simulink model "VCU_CS75_12_27_test_log"  (R2014a)
settings: Solver=FixedStepDiscrete  StartTime=0.0  StopTime=25  FixedStep=0.0005  RelTol=1e-3
undefined symbols (not defined in the file or in its folder): ecucoder_acal, ErrorSumMax1, ErrorSumMax2, ErrorSumMax3, I1, I2, I3, I_SW01_L, LaterlAngleCommand, LDW, Log_ErrorSumMax1, Log_ErrorSumMax2, Log_I1, Log_I2, Log_P1, Log_P2, Log_Takeover, P1, P2, P3, RemoteAcc, RemoteAcclPosition
libraries: simulink x927, ec5744lib x40
(part 24 of 31)

== system VCU_CS75_12_27_test_log/长安CS75底盘程序，20ms一次/Input/CAN0_Rx/a1_211/ReceiveMessages/Subsystem/a1 ==
  input : Inport
  Demux : Demux  Outputs=8
  SCS_Ad : Sum
  SCS_Convert : DataTypeConversion  OutDataTypeStr=uint32
  SCS_F : Gain
  SCS_L : simulink/Logic and Bit Operations/Bitwise Operator  logicop=AND  UseBitMask=on  BitMask=8  BitMaskRealWorld=Stored Integer
  SCS_O : Constant  Value=0  OutDataTypeStr=single
  SCS_S : ArithShift  BitShiftNumber=3
  SCS_Sub : Subsystem
  SCS_sat : Saturate  UpperLimit=1  LowerLimit=0
  SCScv : DataTypeConversion
  Vx_Ad : Sum
  Vx_Convert : DataTypeConversion  OutDataTypeStr=uint32
  Vx_F : Gain  Gain=0.00610360875867857
  Vx_L : simulink/Logic and Bit Operations/Bitwise Operator  logicop=AND  UseBitMask=on  BitMask=65535  BitMaskRealWorld=Stored Integer
  Vx_O : Constant  Value=-200  OutDataTypeStr=single
  Vx_S : ArithShift
  Vx_Sub : Subsystem
  Vx_sat : Saturate  UpperLimit=200  LowerLimit=-200
  Vxcv : DataTypeConversion
  Vxinput8_Ad : Sum
  Vxinput8_C : Constant  Value=256
  Vxinput8_P : Product
  cones_count_actual_Ad : Sum
  cones_count_actual_Convert : DataTypeConversion  OutDataTypeStr=uint32
  cones_count_actual_F : Gain
  cones_count_actual_L : simulink/Logic and Bit Operations/Bitwise Operator  logicop=AND  UseBitMask=on  BitMask=255  BitMaskRealWorld=Stored Integer
  cones_count_actual_O : Constant  Value=0  OutDataTypeStr=single
  cones_count_actual_S : ArithShift
  cones_count_actual_Sub : Subsystem
  cones_count_actual_sat : Saturate  UpperLimit=255  LowerLimit=0
  cones_count_actualcv : DataTypeConversion
  cones_count_all_Ad : Sum
  cones_count_all_Convert : DataTypeConversion  OutDataTypeStr=uint32
  cones_count_all_F : Gain
  cones_count_all_L : simulink/Logic and Bit Operations/Bitwise Operator  logicop=AND  UseBitMask=on  BitMask=255  BitMaskRealWorld=Stored Integer
  cones_count_all_O : Constant  Value=0  OutDataTypeStr=single
  cones_count_all_S : ArithShift
  cones_count_all_Sub : Subsystem
  cones_count_all_sat : Saturate  UpperLimit=255  LowerLimit=0
  cones_count_allcv : DataTypeConversion
  finish_Ad : Sum
  finish_Convert : DataTypeConversion  OutDataTypeStr=uint32
  finish_F : Gain
  finish_L : simulink/Logic and Bit Operations/Bitwise Operator  logicop=AND  UseBitMask=on  BitMask=4  BitMaskRealWorld=Stored Integer
  finish_O : Constant  Value=0  OutDataTypeStr=single
  finish_S : ArithShift  BitShiftNumber=2
  finish_Sub : Subsystem
  finish_sat : Saturate  UpperLimit=1  LowerLimit=0
  finishcv : DataTypeConversion
  mission_Ad : Sum
  mission_Convert : DataTypeConversion  OutDataTypeStr=uint32
  mission_F : Gain
  mission_L : simulink/Logic and Bit Operations/Bitwise Operator  logicop=AND  UseBitMask=on  BitMask=240  BitMaskRealWorld=Stored Integer
  mission_O : Constant  Value=0  OutDataTypeStr=single
  mission_S : ArithShift  BitShiftNumber=4
  mission_Sub : Subsystem
  mission_sat : Saturate  UpperLimit=7  LowerLimit=0
  missioncv : DataTypeConversion
  tap_Ad : Sum
  tap_Convert : DataTypeConversion  OutDataTypeStr=uint32
  tap_F : Gain
  tap_L : simulink/Logic and Bit Operations/Bitwise Operator  logicop=AND  UseBitMask=on  BitMask=3  BitMaskRealWorld=Stored Integer
  tap_O : Constant  Value=0  OutDataTypeStr=single
  tap_S : ArithShift
  tap_Sub : Subsystem
  tap_sat : Saturate  UpperLimit=3  LowerLimit=0
  tapcv : DataTypeConversion
  target_steering_Ad : Sum
  target_steering_Convert : DataTypeConversion  OutDataTypeStr=uint32
  target_steering_F : Gain  Gain=0.0488400488400488
  target_steering_L : simulink/Logic and Bit Operations/Bitwise Operator  logicop=AND  UseBitMask=on  BitMask=4095  BitMaskRealWorld=Stored Integer
  target_steering_O : Constant  Value=-100  OutDataTypeStr=single
  target_steering_S : ArithShift
  target_steering_Sub : Subsystem
  target_steering_sat : Saturate  UpperLimit=99.9999999999998  LowerLimit=-100
  target_steeringcv : DataTypeConversion
  target_steeringinput2_Ad : Sum
  target_steeringinput2_C : Constant  Value=256
  target_steeringinput2_P : Product
  throttlevbrake_position_Ad : Sum
  throttlevbrake_position_Convert : DataTypeConversion  OutDataTypeStr=uint32
  throttlevbrake_position_F : Gain  Gain=0.0488400488400488
  throttlevbrake_position_L : simulink/Logic and Bit Operations/Bitwise Operator  logicop=AND  UseBitMask=on  BitMask=65520  BitMaskRealWorld=Stored Integer
  throttlevbrake_position_O : Constant  Value=-100  OutDataTypeStr=single
  throttlevbrake_position_S : ArithShift  BitShiftNumber=4
  throttlevbrake_position_Sub : Subsystem
  throttlevbrake_position_sat : Saturate  UpperLimit=100  LowerLimit=-100
  throttlevbrake_positioncv : DataTypeConversion
  throttlevbrake_positioninput3_Ad : Sum
  throttlevbrake_positioninput3_C : Constant  Value=256
  throttlevbrake_positioninput3_P : Product
  Vx_Out : Outport
  mission_Out : Outport  Port=2
  SCS_Out : Outport  Port=3
  finish_Out : Outport  Port=4
  tap_Out : Outport  Port=5
  cones_count_all_Out : Outport  Port=6
  cones_count_actual_Out : Outport  Port=7
  throttlevbrake_position_Out : Outport  Port=8
  target_steering_Out : Outport  Port=9
  wires:
  Vx_F/1 -> Vx_Ad/1
  Vx_O/1 -> Vx_Ad/2
  Vx_Ad/1 -> Vx_sat/1
  Vx_sat/1 -> Vx_Out/1
  Demux/8 -> Vxinput8_P/1
  Vxinput8_C/1 -> Vxinput8_P/2
  Vxinput8_P/1 -> Vxinput8_Ad/1
  Demux/7 -> Vxinput8_Ad/2
  Vxinput8_Ad/1 -> Vx_Sub/1(In1)
  Vx_Sub/1(Out1) -> Vx_Convert/1
  Vx_Convert/1 -> Vx_L/1
  Vx_L/1 -> Vx_S/1
  Vx_S/1 -> Vxcv/1
  Vxcv/1 -> Vx_F/1
  mission_F/1 -> mission_Ad/1
  mission_O/1 -> mission_Ad/2
  mission_Ad/1 -> mission_sat/1
  mission_sat/1 -> mission_Out/1
  Demux/6 -> mission_Sub/1(In1), SCS_Sub/1(In1), finish_Sub/1(In1), tap_Sub/1(In1)
  mission_Sub/1(Out1) -> mission_Convert/1
  mission_Convert/1 -> mission_L/1
  mission_L/1 -> mission_S/1
  mission_S/1 -> missioncv/1
  missioncv/1 -> mission_F/1
  SCS_F/1 -> SCS_Ad/1
  SCS_O/1 -> SCS_Ad/2
  SCS_Ad/1 -> SCS_sat/1
  SCS_sat/1 -> SCS_Out/1
  SCS_Sub/1(Out1) -> SCS_Convert/1
  SCS_Convert/1 -> SCS_L/1
  SCS_L/1 -> SCS_S/1
  SCS_S/1 -> SCScv/1
  SCScv/1 -> SCS_F/1
  finish_F/1 -> finish_Ad/1
  finish_O/1 -> finish_Ad/2
  finish_Ad/1 -> finish_sat/1
  finish_sat/1 -> finish_Out/1
  finish_Sub/1(Out1) -> finish_Convert/1
  finish_Convert/1 -> finish_L/1
  finish_L/1 -> finish_S/1
  finish_S/1 -> finishcv/1
  finishcv/1 -> finish_F/1
  tap_F/1 -> tap_Ad/1
  tap_O/1 -> tap_Ad/2
  tap_Ad/1 -> tap_sat/1
  tap_sat/1 -> tap_Out/1
  tap_Sub/1(Out1) -> tap_Convert/1
  tap_Convert/1 -> tap_L/1
  tap_L/1 -> tap_S/1
  tap_S/1 -> tapcv/1
  tapcv/1 -> tap_F/1
  cones_count_all_F/1 -> cones_count_all_Ad/1
  cones_count_all_O/1 -> cones_count_all_Ad/2
  cones_count_all_Ad/1 -> cones_count_all_sat/1
  cones_count_all_sat/1 -> cones_count_all_Out/1
  Demux/5 -> cones_count_all_Sub/1(In1)
  cones_count_all_Sub/1(Out1) -> cones_count_all_Convert/1
  cones_count_all_Convert/1 -> cones_count_all_L/1
  cones_count_all_L/1 -> cones_count_all_S/1
  cones_count_all_S/1 -> cones_count_allcv/1
  cones_count_allcv/1 -> cones_count_all_F/1
  cones_count_actual_F/1 -> cones_count_actual_Ad/1
  cones_count_actual_O/1 -> cones_count_actual_Ad/2
  cones_count_actual_Ad/1 -> cones_count_actual_sat/1
  cones_count_actual_sat/1 -> cones_count_actual_Out/1
  Demux/4 -> cones_count_actual_Sub/1(In1)
  cones_count_actual_Sub/1(Out1) -> cones_count_actual_Convert/1
  cones_count_actual_Convert/1 -> cones_count_actual_L/1
  cones_count_actual_L/1 -> cones_count_actual_S/1
  cones_count_actual_S/1 -> cones_count_actualcv/1
  cones_count_actualcv/1 -> cones_count_actual_F/1
  throttlevbrake_position_F/1 -> throttlevbrake_position_Ad/1
  throttlevbrake_position_O/1 -> throttlevbrake_position_Ad/2
  throttlevbrake_position_Ad/1 -> throttlevbrake_position_sat/1
  throttlevbrake_position_sat/1 -> throttlevbrake_position_Out/1
  Demux/3 -> throttlevbrake_positioninput3_P/1
  throttlevbrake_positioninput3_C/1 -> throttlevbrake_positioninput3_P/2
  throttlevbrake_positioninput3_P/1 -> throttlevbrake_positioninput3_Ad/1
  Demux/2 -> throttlevbrake_positioninput3_Ad/2, target_steeringinput2_P/1
  throttlevbrake_positioninput3_Ad/1 -> throttlevbrake_position_Sub/1(In1)
  throttlevbrake_position_Sub/1(Out1) -> throttlevbrake_position_Convert/1
  throttlevbrake_position_Convert/1 -> throttlevbrake_position_L/1
  throttlevbrake_position_L/1 -> throttlevbrake_position_S/1
  throttlevbrake_position_S/1 -> throttlevbrake_positioncv/1
  throttlevbrake_positioncv/1 -> throttlevbrake_position_F/1
  target_steering_F/1 -> target_steering_Ad/1
  target_steering_O/1 -> target_steering_Ad/2
  target_steering_Ad/1 -> target_steering_sat/1
  target_steering_sat/1 -> target_steering_Out/1
  target_steeringinput2_C/1 -> target_steeringinput2_P/2
  target_steeringinput2_P/1 -> target_steeringinput2_Ad/1
  Demux/1 -> target_steeringinput2_Ad/2
  target_steeringinput2_Ad/1 -> target_steering_Sub/1(In1)
  target_steering_Sub/1(Out1) -> target_steering_Convert/1
  target_steering_Convert/1 -> target_steering_L/1
  target_steering_L/1 -> target_steering_S/1
  target_steering_S/1 -> target_steeringcv/1
  target_steeringcv/1 -> target_steering_F/1
  input/1 -> Demux/1

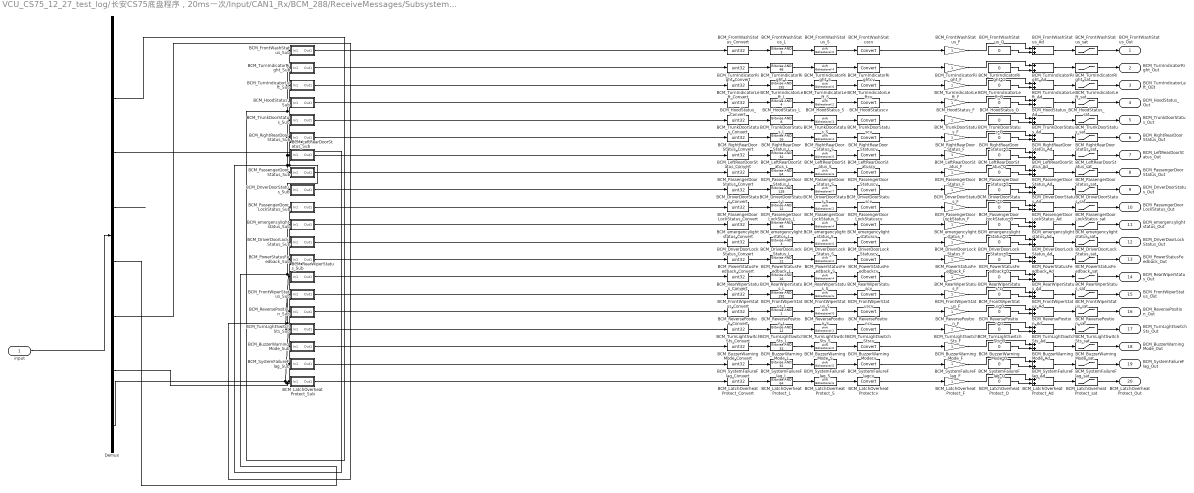
== system VCU_CS75_12_27_test_log/长安CS75底盘程序，20ms一次/Input/CAN1_Rx/BCM_288/ReceiveMessages/Subsystem/BCM_1 ==
  input : Inport
  BCM_BuzzerWarningMode_Ad : Sum
  BCM_BuzzerWarningMode_Convert : DataTypeConversion  OutDataTypeStr=uint32
  BCM_BuzzerWarningMode_F : Gain
  BCM_BuzzerWarningMode_L : simulink/Logic and Bit Operations/Bitwise Operator  logicop=AND  UseBitMask=on  BitMask=31  BitMaskRealWorld=Stored Integer
  BCM_BuzzerWarningMode_O : Constant  Value=0  OutDataTypeStr=single
  BCM_BuzzerWarningMode_S : ArithShift
  BCM_BuzzerWarningMode_Sub : Subsystem
  BCM_BuzzerWarningMode_sat : Saturate  UpperLimit=31  LowerLimit=0
  BCM_BuzzerWarningModecv : DataTypeConversion
  BCM_DriverDoorLockStatus_Ad : Sum
  BCM_DriverDoorLockStatus_Convert : DataTypeConversion  OutDataTypeStr=uint32
  BCM_DriverDoorLockStatus_F : Gain
  BCM_DriverDoorLockStatus_L : simulink/Logic and Bit Operations/Bitwise Operator  logicop=AND  UseBitMask=on  BitMask=3  BitMaskRealWorld=Stored Integer
  BCM_DriverDoorLockStatus_O : Constant  Value=0  OutDataTypeStr=single
  BCM_DriverDoorLockStatus_S : ArithShift
  BCM_DriverDoorLockStatus_Sub : Subsystem
  BCM_DriverDoorLockStatus_sat : Saturate  UpperLimit=3  LowerLimit=0
  BCM_DriverDoorLockStatuscv : DataTypeConversion
  BCM_DriverDoorStatus_Ad : Sum
  BCM_DriverDoorStatus_Convert : DataTypeConversion  OutDataTypeStr=uint32
  BCM_DriverDoorStatus_F : Gain
  BCM_DriverDoorStatus_L : simulink/Logic and Bit Operations/Bitwise Operator  logicop=AND  UseBitMask=on  BitMask=128  BitMaskRealWorld=Stored Integer
  BCM_DriverDoorStatus_O : Constant  Value=0  OutDataTypeStr=single
  BCM_DriverDoorStatus_S : ArithShift  BitShiftNumber=7
  BCM_DriverDoorStatus_Sub : Subsystem
  BCM_DriverDoorStatus_sat : Saturate  UpperLimit=1  LowerLimit=0
  BCM_DriverDoorStatuscv : DataTypeConversion
  BCM_FrontWashStatus_Ad : Sum
  BCM_FrontWashStatus_Convert : DataTypeConversion  OutDataTypeStr=uint32
  BCM_FrontWashStatus_F : Gain
  BCM_FrontWashStatus_L : simulink/Logic and Bit Operations/Bitwise Operator  logicop=AND  UseBitMask=on  BitMask=3  BitMaskRealWorld=Stored Integer
  BCM_FrontWashStatus_O : Constant  Value=0  OutDataTypeStr=single
  BCM_FrontWashStatus_S : ArithShift
  BCM_FrontWashStatus_Sub : Subsystem
  BCM_FrontWashStatus_sat : Saturate  UpperLimit=3  LowerLimit=0
  BCM_FrontWashStatuscv : DataTypeConversion
  BCM_FrontWiperStatus_Ad : Sum
  BCM_FrontWiperStatus_Convert : DataTypeConversion  OutDataTypeStr=uint32
  BCM_FrontWiperStatus_F : Gain
  BCM_FrontWiperStatus_L : simulink/Logic and Bit Operations/Bitwise Operator  logicop=AND  UseBitMask=on  BitMask=192  BitMaskRealWorld=Stored Integer
  BCM_FrontWiperStatus_O : Constant  Value=0  OutDataTypeStr=single
  BCM_FrontWiperStatus_S : ArithShift  BitShiftNumber=6
  BCM_FrontWiperStatus_Sub : Subsystem
  BCM_FrontWiperStatus_sat : Saturate  UpperLimit=3  LowerLimit=0
  BCM_FrontWiperStatuscv : DataTypeConversion
  BCM_HoodStatus_Ad : Sum
  BCM_HoodStatus_Convert : DataTypeConversion  OutDataTypeStr=uint32
  BCM_HoodStatus_F : Gain
  BCM_HoodStatus_L : simulink/Logic and Bit Operations/Bitwise Operator  logicop=AND  UseBitMask=on  BitMask=4  BitMaskRealWorld=Stored Integer
  BCM_HoodStatus_O : Constant  Value=0  OutDataTypeStr=single
  BCM_HoodStatus_S : ArithShift  BitShiftNumber=2
  BCM_HoodStatus_Sub : Subsystem
  BCM_HoodStatus_sat : Saturate  UpperLimit=1  LowerLimit=0
  BCM_HoodStatuscv : DataTypeConversion
  BCM_LatchOverheatProtect_Ad : Sum
  BCM_LatchOverheatProtect_Convert : DataTypeConversion  OutDataTypeStr=uint32
  BCM_LatchOverheatProtect_F : Gain
  BCM_LatchOverheatProtect_L : simulink/Logic and Bit Operations/Bitwise Operator  logicop=AND  UseBitMask=on  BitMask=64  BitMaskRealWorld=Stored Integer
  BCM_LatchOverheatProtect_O : Constant  Value=0  OutDataTypeStr=single
  BCM_LatchOverheatProtect_S : ArithShift  BitShiftNumber=6
  BCM_LatchOverheatProtect_Sub : Subsystem
  BCM_LatchOverheatProtect_sat : Saturate  UpperLimit=1  LowerLimit=0
  BCM_LatchOverheatProtectcv : DataTypeConversion
  BCM_LeftRearDoorStatus_Ad : Sum
  BCM_LeftRearDoorStatus_Convert : DataTypeConversion  OutDataTypeStr=uint32
  BCM_LeftRearDoorStatus_F : Gain
  BCM_LeftRearDoorStatus_L : simulink/Logic and Bit Operations/Bitwise Operator  logicop=AND  UseBitMask=on  BitMask=32  BitMaskRealWorld=Stored Integer
  BCM_LeftRearDoorStatus_O : Constant  Value=0  OutDataTypeStr=single
  BCM_LeftRearDoorStatus_S : ArithShift  BitShiftNumber=5
  BCM_LeftRearDoorStatus_Sub : Subsystem
  BCM_LeftRearDoorStatus_sat : Saturate  UpperLimit=1  LowerLimit=0
  BCM_LeftRearDoorStatuscv : DataTypeConversion
  BCM_PassengerDoorLockStatus_Ad : Sum
  BCM_PassengerDoorLockStatus_Convert : DataTypeConversion  OutDataTypeStr=uint32
  BCM_PassengerDoorLockStatus_F : Gain
  BCM_PassengerDoorLockStatus_L : simulink/Logic and Bit Operations/Bitwise Operator  logicop=AND  UseBitMask=on  BitMask=12  BitMaskRealWorld=Stored Integer
  BCM_PassengerDoorLockStatus_O : Constant  Value=0  OutDataTypeStr=single
  BCM_PassengerDoorLockStatus_S : ArithShift  BitShiftNumber=2
  BCM_PassengerDoorLockStatus_Sub : Subsystem
  BCM_PassengerDoorLockStatus_sat : Saturate  UpperLimit=3  LowerLimit=0
  BCM_PassengerDoorLockStatuscv : DataTypeConversion
  BCM_PassengerDoorStatus_Ad : Sum
  BCM_PassengerDoorStatus_Convert : DataTypeConversion  OutDataTypeStr=uint32
  BCM_PassengerDoorStatus_F : Gain
  BCM_PassengerDoorStatus_L : simulink/Logic and Bit Operations/Bitwise Operator  logicop=AND  UseBitMask=on  BitMask=64  BitMaskRealWorld=Stored Integer
  BCM_PassengerDoorStatus_O : Constant  Value=0  OutDataTypeStr=single
  BCM_PassengerDoorStatus_S : ArithShift  BitShiftNumber=6
  BCM_PassengerDoorStatus_Sub : Subsystem
  BCM_PassengerDoorStatus_sat : Saturate  UpperLimit=1  LowerLimit=0
  BCM_PassengerDoorStatuscv : DataTypeConversion
  BCM_PowerStatusFeedback_Ad : Sum
  BCM_PowerStatusFeedback_Convert : DataTypeConversion  OutDataTypeStr=uint32
  BCM_PowerStatusFeedback_F : Gain
  BCM_PowerStatusFeedback_L : simulink/Logic and Bit Operations/Bitwise Operator  logicop=AND  UseBitMask=on  BitMask=12  BitMaskRealWorld=Stored Integer
  BCM_PowerStatusFeedback_O : Constant  Value=0  OutDataTypeStr=single
  BCM_PowerStatusFeedback_S : ArithShift  BitShiftNumber=2
  BCM_PowerStatusFeedback_Sub : Subsystem
  BCM_PowerStatusFeedback_sat : Saturate  UpperLimit=3  LowerLimit=0
  BCM_PowerStatusFeedbackcv : DataTypeConversion
  BCM_RearWiperStatus_Ad : Sum
  BCM_RearWiperStatus_Convert : DataTypeConversion  OutDataTypeStr=uint32
  BCM_RearWiperStatus_F : Gain
  BCM_RearWiperStatus_L : simulink/Logic and Bit Operations/Bitwise Operator  logicop=AND  UseBitMask=on  BitMask=16  BitMaskRealWorld=Stored Integer
  BCM_RearWiperStatus_O : Constant  Value=0  OutDataTypeStr=single
  BCM_RearWiperStatus_S : ArithShift  BitShiftNumber=4
  BCM_RearWiperStatus_Sub : Subsystem
  BCM_RearWiperStatus_sat : Saturate  UpperLimit=1  LowerLimit=0
  BCM_RearWiperStatuscv : DataTypeConversion
  BCM_ReversePosition_Ad : Sum
  BCM_ReversePosition_Convert : DataTypeConversion  OutDataTypeStr=uint32
  BCM_ReversePosition_F : Gain
  BCM_ReversePosition_L : simulink/Logic and Bit Operations/Bitwise Operator  logicop=AND  UseBitMask=on  BitMask=1  BitMaskRealWorld=Stored Integer
  BCM_ReversePosition_O : Constant  Value=0  OutDataTypeStr=single
  BCM_ReversePosition_S : ArithShift
  BCM_ReversePosition_Sub : Subsystem
  BCM_ReversePosition_sat : Saturate  UpperLimit=1  LowerLimit=0
  BCM_ReversePositioncv : DataTypeConversion
  BCM_RightRearDoorStatus_Ad : Sum
  BCM_RightRearDoorStatus_Convert : DataTypeConversion  OutDataTypeStr=uint32
  BCM_RightRearDoorStatus_F : Gain
  BCM_RightRearDoorStatus_L : simulink/Logic and Bit Operations/Bitwise Operator  logicop=AND  UseBitMask=on  BitMask=16  BitMaskRealWorld=Stored Integer
  BCM_RightRearDoorStatus_O : Constant  Value=0  OutDataTypeStr=single
  BCM_RightRearDoorStatus_S : ArithShift  BitShiftNumber=4
  BCM_RightRearDoorStatus_Sub : Subsystem
  BCM_RightRearDoorStatus_sat : Saturate  UpperLimit=1  LowerLimit=0
  BCM_RightRearDoorStatuscv : DataTypeConversion
  BCM_SystemFailureFlag_Ad : Sum
  BCM_SystemFailureFlag_Convert : DataTypeConversion  OutDataTypeStr=uint32
  BCM_SystemFailureFlag_F : Gain
  BCM_SystemFailureFlag_L : simulink/Logic and Bit Operations/Bitwise Operator  logicop=AND  UseBitMask=on  BitMask=32  BitMaskRealWorld=Stored Integer
  BCM_SystemFailureFlag_O : Constant  Value=0  OutDataTypeStr=single
  BCM_SystemFailureFlag_S : ArithShift  BitShiftNumber=5
  BCM_SystemFailureFlag_Sub : Subsystem
  BCM_SystemFailureFlag_sat : Saturate  UpperLimit=1  LowerLimit=0
  BCM_SystemFailureFlagcv : DataTypeConversion
  BCM_TrunkDoorStatus_Ad : Sum
  BCM_TrunkDoorStatus_Convert : DataTypeConversion  OutDataTypeStr=uint32
  BCM_TrunkDoorStatus_F : Gain
  BCM_TrunkDoorStatus_L : simulink/Logic and Bit Operations/Bitwise Operator  logicop=AND  UseBitMask=on  BitMask=8  BitMaskRealWorld=Stored Integer
  BCM_TrunkDoorStatus_O : Constant  Value=0  OutDataTypeStr=single
  BCM_TrunkDoorStatus_S : ArithShift  BitShiftNumber=3
  BCM_TrunkDoorStatus_Sub : Subsystem
  BCM_TrunkDoorStatus_sat : Saturate  UpperLimit=1  LowerLimit=0
  BCM_TrunkDoorStatuscv : DataTypeConversion
  BCM_TurnIndicatorLeft_Ad : Sum
  BCM_TurnIndicatorLeft_Convert : DataTypeConversion  OutDataTypeStr=uint32
  BCM_TurnIndicatorLeft_F : Gain
  BCM_TurnIndicatorLeft_L : simulink/Logic and Bit Operations/Bitwise Operator  logicop=AND  UseBitMask=on  BitMask=192  BitMaskRealWorld=Stored Integer
  BCM_TurnIndicatorLeft_O : Constant  Value=0  OutDataTypeStr=single
  BCM_TurnIndicatorLeft_S : ArithShift  BitShiftNumber=6
  BCM_TurnIndicatorLeft_Sub : Subsystem
  BCM_TurnIndicatorLeft_sat : Saturate  UpperLimit=3  LowerLimit=0
  BCM_TurnIndicatorLeftcv : DataTypeConversion
  BCM_TurnIndicatorRight_Ad : Sum
  BCM_TurnIndicatorRight_Convert : DataTypeConversion  OutDataTypeStr=uint32
  BCM_TurnIndicatorRight_F : Gain
  BCM_TurnIndicatorRight_L : simulink/Logic and Bit Operations/Bitwise Operator  logicop=AND  UseBitMask=on  BitMask=48  BitMaskRealWorld=Stored Integer
  BCM_TurnIndicatorRight_O : Constant  Value=0  OutDataTypeStr=single
  BCM_TurnIndicatorRight_S : ArithShift  BitShiftNumber=4
  BCM_TurnIndicatorRight_Sub : Subsystem
  BCM_TurnIndicatorRight_sat : Saturate  UpperLimit=3  LowerLimit=0
  BCM_TurnIndicatorRightcv : DataTypeConversion
  BCM_TurnLightSwitchSts_Ad : Sum
  BCM_TurnLightSwitchSts_Convert : DataTypeConversion  OutDataTypeStr=uint32
  BCM_TurnLightSwitchSts_F : Gain
  BCM_TurnLightSwitchSts_L : simulink/Logic and Bit Operations/Bitwise Operator  logicop=AND  UseBitMask=on  BitMask=12  BitMaskRealWorld=Stored Integer
  BCM_TurnLightSwitchSts_O : Constant  Value=0  OutDataTypeStr=single
  BCM_TurnLightSwitchSts_S : ArithShift  BitShiftNumber=2
  BCM_TurnLightSwitchSts_Sub : Subsystem
  BCM_TurnLightSwitchSts_sat : Saturate  UpperLimit=3  LowerLimit=0
  BCM_TurnLightSwitchStscv : DataTypeConversion
  BCM_emergencylightstatus_Ad : Sum
  BCM_emergencylightstatus_Convert : DataTypeConversion  OutDataTypeStr=uint32
  BCM_emergencylightstatus_F : Gain
  BCM_emergencylightstatus_L : simulink/Logic and Bit Operations/Bitwise Operator  logicop=AND  UseBitMask=on  BitMask=48  BitMaskRealWorld=Stored Integer
  BCM_emergencylightstatus_O : Constant  Value=0  OutDataTypeStr=single
  BCM_emergencylightstatus_S : ArithShift  BitShiftNumber=4
  BCM_emergencylightstatus_Sub : Subsystem
  BCM_emergencylightstatus_sat : Saturate  UpperLimit=3  LowerLimit=0
  BCM_emergencylightstatuscv : DataTypeConversion
  Demux : Demux  Outputs=8
  BCM_FrontWashStatus_Out : Outport
  BCM_TurnIndicatorRight_Out : Outport  Port=2
  BCM_TurnIndicatorLeft_Out : Outport  Port=3
  BCM_HoodStatus_Out : Outport  Port=4
  BCM_TrunkDoorStatus_Out : Outport  Port=5
  BCM_RightRearDoorStatus_Out : Outport  Port=6
  BCM_LeftRearDoorStatus_Out : Outport  Port=7
  BCM_PassengerDoorStatus_Out : Outport  Port=8
  BCM_DriverDoorStatus_Out : Outport  Port=9
  BCM_PassengerDoorLockStatus_Out : Outport  Port=10
  BCM_emergencylightstatus_Out : Outport  Port=11
  BCM_DriverDoorLockStatus_Out : Outport  Port=12
  BCM_PowerStatusFeedback_Out : Outport  Port=13
  BCM_RearWiperStatus_Out : Outport  Port=14
  BCM_FrontWiperStatus_Out : Outport  Port=15
  BCM_ReversePosition_Out : Outport  Port=16
  BCM_TurnLightSwitchSts_Out : Outport  Port=17
  BCM_BuzzerWarningMode_Out : Outport  Port=18
  BCM_SystemFailureFlag_Out : Outport  Port=19
  BCM_LatchOverheatProtect_Out : Outport  Port=20
  wires:
  input/1 -> Demux/1
  BCM_LatchOverheatProtectcv/1 -> BCM_LatchOverheatProtect_F/1
  BCM_LatchOverheatProtect_S/1 -> BCM_LatchOverheatProtectcv/1
  BCM_LatchOverheatProtect_L/1 -> BCM_LatchOverheatProtect_S/1
  BCM_LatchOverheatProtect_Convert/1 -> BCM_LatchOverheatProtect_L/1
  BCM_LatchOverheatProtect_Sub/1(Out1) -> BCM_LatchOverheatProtect_Convert/1
  BCM_LatchOverheatProtect_sat/1 -> BCM_LatchOverheatProtect_Out/1
  BCM_LatchOverheatProtect_Ad/1 -> BCM_LatchOverheatProtect_sat/1
  BCM_LatchOverheatProtect_O/1 -> BCM_LatchOverheatProtect_Ad/2
  BCM_LatchOverheatProtect_F/1 -> BCM_LatchOverheatProtect_Ad/1
  BCM_SystemFailureFlagcv/1 -> BCM_SystemFailureFlag_F/1
  BCM_SystemFailureFlag_S/1 -> BCM_SystemFailureFlagcv/1
  BCM_SystemFailureFlag_L/1 -> BCM_SystemFailureFlag_S/1
  BCM_SystemFailureFlag_Convert/1 -> BCM_SystemFailureFlag_L/1
  BCM_SystemFailureFlag_Sub/1(Out1) -> BCM_SystemFailureFlag_Convert/1
  BCM_SystemFailureFlag_sat/1 -> BCM_SystemFailureFlag_Out/1
  BCM_SystemFailureFlag_Ad/1 -> BCM_SystemFailureFlag_sat/1
  BCM_SystemFailureFlag_O/1 -> BCM_SystemFailureFlag_Ad/2
  BCM_SystemFailureFlag_F/1 -> BCM_SystemFailureFlag_Ad/1
  BCM_BuzzerWarningModecv/1 -> BCM_BuzzerWarningMode_F/1
  BCM_BuzzerWarningMode_S/1 -> BCM_BuzzerWarningModecv/1
  BCM_BuzzerWarningMode_L/1 -> BCM_BuzzerWarningMode_S/1
  BCM_BuzzerWarningMode_Convert/1 -> BCM_BuzzerWarningMode_L/1
  BCM_BuzzerWarningMode_Sub/1(Out1) -> BCM_BuzzerWarningMode_Convert/1
  Demux/8 -> BCM_SystemFailureFlag_Sub/1(In1), BCM_BuzzerWarningMode_Sub/1(In1), BCM_LatchOverheatProtect_Sub/1(In1)
  BCM_BuzzerWarningMode_sat/1 -> BCM_BuzzerWarningMode_Out/1
  BCM_BuzzerWarningMode_Ad/1 -> BCM_BuzzerWarningMode_sat/1
  BCM_BuzzerWarningMode_O/1 -> BCM_BuzzerWarningMode_Ad/2
  BCM_BuzzerWarningMode_F/1 -> BCM_BuzzerWarningMode_Ad/1
  BCM_TurnLightSwitchStscv/1 -> BCM_TurnLightSwitchSts_F/1
  BCM_TurnLightSwitchSts_S/1 -> BCM_TurnLightSwitchStscv/1
  BCM_TurnLightSwitchSts_L/1 -> BCM_TurnLightSwitchSts_S/1
  BCM_TurnLightSwitchSts_Convert/1 -> BCM_TurnLightSwitchSts_L/1
  BCM_TurnLightSwitchSts_Sub/1(Out1) -> BCM_TurnLightSwitchSts_Convert/1
  BCM_TurnLightSwitchSts_sat/1 -> BCM_TurnLightSwitchSts_Out/1
  BCM_TurnLightSwitchSts_Ad/1 -> BCM_TurnLightSwitchSts_sat/1
  BCM_TurnLightSwitchSts_O/1 -> BCM_TurnLightSwitchSts_Ad/2
  BCM_TurnLightSwitchSts_F/1 -> BCM_TurnLightSwitchSts_Ad/1
  BCM_ReversePositioncv/1 -> BCM_ReversePosition_F/1
  BCM_ReversePosition_S/1 -> BCM_ReversePositioncv/1
  BCM_ReversePosition_L/1 -> BCM_ReversePosition_S/1
  BCM_ReversePosition_Convert/1 -> BCM_ReversePosition_L/1
  BCM_ReversePosition_Sub/1(Out1) -> BCM_ReversePosition_Convert/1
  Demux/7 -> BCM_TurnLightSwitchSts_Sub/1(In1), BCM_ReversePosition_Sub/1(In1)
  BCM_ReversePosition_sat/1 -> BCM_ReversePosition_Out/1
  BCM_ReversePosition_Ad/1 -> BCM_ReversePosition_sat/1
  BCM_ReversePosition_O/1 -> BCM_ReversePosition_Ad/2
  BCM_ReversePosition_F/1 -> BCM_ReversePosition_Ad/1
  BCM_FrontWiperStatuscv/1 -> BCM_FrontWiperStatus_F/1
  BCM_FrontWiperStatus_S/1 -> BCM_FrontWiperStatuscv/1
  BCM_FrontWiperStatus_L/1 -> BCM_FrontWiperStatus_S/1
  BCM_FrontWiperStatus_Convert/1 -> BCM_FrontWiperStatus_L/1
  BCM_FrontWiperStatus_Sub/1(Out1) -> BCM_FrontWiperStatus_Convert/1
  BCM_FrontWiperStatus_sat/1 -> BCM_FrontWiperStatus_Out/1
  BCM_FrontWiperStatus_Ad/1 -> BCM_FrontWiperStatus_sat/1
  BCM_FrontWiperStatus_O/1 -> BCM_FrontWiperStatus_Ad/2
  BCM_FrontWiperStatus_F/1 -> BCM_FrontWiperStatus_Ad/1
  BCM_RearWiperStatuscv/1 -> BCM_RearWiperStatus_F/1
  BCM_RearWiperStatus_S/1 -> BCM_RearWiperStatuscv/1
  BCM_RearWiperStatus_L/1 -> BCM_RearWiperStatus_S/1
  BCM_RearWiperStatus_Convert/1 -> BCM_RearWiperStatus_L/1
  BCM_RearWiperStatus_Sub/1(Out1) -> BCM_RearWiperStatus_Convert/1
  BCM_RearWiperStatus_sat/1 -> BCM_RearWiperStatus_Out/1
  BCM_RearWiperStatus_Ad/1 -> BCM_RearWiperStatus_sat/1
  BCM_RearWiperStatus_O/1 -> BCM_RearWiperStatus_Ad/2
  BCM_RearWiperStatus_F/1 -> BCM_RearWiperStatus_Ad/1
  BCM_PowerStatusFeedbackcv/1 -> BCM_PowerStatusFeedback_F/1
  BCM_PowerStatusFeedback_S/1 -> BCM_PowerStatusFeedbackcv/1
  BCM_PowerStatusFeedback_L/1 -> BCM_PowerStatusFeedback_S/1
  BCM_PowerStatusFeedback_Convert/1 -> BCM_PowerStatusFeedback_L/1
  BCM_PowerStatusFeedback_Sub/1(Out1) -> BCM_PowerStatusFeedback_Convert/1
  BCM_PowerStatusFeedback_sat/1 -> BCM_PowerStatusFeedback_Out/1
  BCM_PowerStatusFeedback_Ad/1 -> BCM_PowerStatusFeedback_sat/1
  BCM_PowerStatusFeedback_O/1 -> BCM_PowerStatusFeedback_Ad/2
  BCM_PowerStatusFeedback_F/1 -> BCM_PowerStatusFeedback_Ad/1
  BCM_DriverDoorLockStatuscv/1 -> BCM_DriverDoorLockStatus_F/1
  BCM_DriverDoorLockStatus_S/1 -> BCM_DriverDoorLockStatuscv/1
  BCM_DriverDoorLockStatus_L/1 -> BCM_DriverDoorLockStatus_S/1
  BCM_DriverDoorLockStatus_Convert/1 -> BCM_DriverDoorLockStatus_L/1
  BCM_DriverDoorLockStatus_Sub/1(Out1) -> BCM_DriverDoorLockStatus_Convert/1
  Demux/6 -> BCM_PowerStatusFeedback_Sub/1(In1), BCM_DriverDoorLockStatus_Sub/1(In1), BCM_RearWiperStatus_Sub/1(In1), BCM_FrontWiperStatus_Sub/1(In1)
  BCM_DriverDoorLockStatus_sat/1 -> BCM_DriverDoorLockStatus_Out/1
  BCM_DriverDoorLockStatus_Ad/1 -> BCM_DriverDoorLockStatus_sat/1
  BCM_DriverDoorLockStatus_O/1 -> BCM_DriverDoorLockStatus_Ad/2
  BCM_DriverDoorLockStatus_F/1 -> BCM_DriverDoorLockStatus_Ad/1
  BCM_emergencylightstatuscv/1 -> BCM_emergencylightstatus_F/1
  BCM_emergencylightstatus_S/1 -> BCM_emergencylightstatuscv/1
  BCM_emergencylightstatus_L/1 -> BCM_emergencylightstatus_S/1
  BCM_emergencylightstatus_Convert/1 -> BCM_emergencylightstatus_L/1
  BCM_emergencylightstatus_Sub/1(Out1) -> BCM_emergencylightstatus_Convert/1
  BCM_emergencylightstatus_sat/1 -> BCM_emergencylightstatus_Out/1
  BCM_emergencylightstatus_Ad/1 -> BCM_emergencylightstatus_sat/1
  BCM_emergencylightstatus_O/1 -> BCM_emergencylightstatus_Ad/2
  BCM_emergencylightstatus_F/1 -> BCM_emergencylightstatus_Ad/1
  BCM_PassengerDoorLockStatuscv/1 -> BCM_PassengerDoorLockStatus_F/1
  BCM_PassengerDoorLockStatus_S/1 -> BCM_PassengerDoorLockStatuscv/1
  BCM_PassengerDoorLockStatus_L/1 -> BCM_PassengerDoorLockStatus_S/1
  BCM_PassengerDoorLockStatus_Convert/1 -> BCM_PassengerDoorLockStatus_L/1
  BCM_PassengerDoorLockStatus_Sub/1(Out1) -> BCM_PassengerDoorLockStatus_Convert/1
  Demux/5 -> BCM_emergencylightstatus_Sub/1(In1), BCM_PassengerDoorLockStatus_Sub/1(In1)
  BCM_PassengerDoorLockStatus_sat/1 -> BCM_PassengerDoorLockStatus_Out/1
  BCM_PassengerDoorLockStatus_Ad/1 -> BCM_PassengerDoorLockStatus_sat/1
  BCM_PassengerDoorLockStatus_O/1 -> BCM_PassengerDoorLockStatus_Ad/2
  BCM_PassengerDoorLockStatus_F/1 -> BCM_PassengerDoorLockStatus_Ad/1
  BCM_DriverDoorStatuscv/1 -> BCM_DriverDoorStatus_F/1
  BCM_DriverDoorStatus_S/1 -> BCM_DriverDoorStatuscv/1
  BCM_DriverDoorStatus_L/1 -> BCM_DriverDoorStatus_S/1
  BCM_DriverDoorStatus_Convert/1 -> BCM_DriverDoorStatus_L/1
  BCM_DriverDoorStatus_Sub/1(Out1) -> BCM_DriverDoorStatus_Convert/1
  BCM_DriverDoorStatus_sat/1 -> BCM_DriverDoorStatus_Out/1
  BCM_DriverDoorStatus_Ad/1 -> BCM_DriverDoorStatus_sat/1
  BCM_DriverDoorStatus_O/1 -> BCM_DriverDoorStatus_Ad/2
  BCM_DriverDoorStatus_F/1 -> BCM_DriverDoorStatus_Ad/1
  BCM_PassengerDoorStatuscv/1 -> BCM_PassengerDoorStatus_F/1
  BCM_PassengerDoorStatus_S/1 -> BCM_PassengerDoorStatuscv/1
  BCM_PassengerDoorStatus_L/1 -> BCM_PassengerDoorStatus_S/1
  BCM_PassengerDoorStatus_Convert/1 -> BCM_PassengerDoorStatus_L/1
  BCM_PassengerDoorStatus_Sub/1(Out1) -> BCM_PassengerDoorStatus_Convert/1
  BCM_PassengerDoorStatus_sat/1 -> BCM_PassengerDoorStatus_Out/1
  BCM_PassengerDoorStatus_Ad/1 -> BCM_PassengerDoorStatus_sat/1
  BCM_PassengerDoorStatus_O/1 -> BCM_PassengerDoorStatus_Ad/2
  BCM_PassengerDoorStatus_F/1 -> BCM_PassengerDoorStatus_Ad/1
  BCM_LeftRearDoorStatuscv/1 -> BCM_LeftRearDoorStatus_F/1
  BCM_LeftRearDoorStatus_S/1 -> BCM_LeftRearDoorStatuscv/1
  BCM_LeftRearDoorStatus_L/1 -> BCM_LeftRearDoorStatus_S/1
  BCM_LeftRearDoorStatus_Convert/1 -> BCM_LeftRearDoorStatus_L/1
  BCM_LeftRearDoorStatus_Sub/1(Out1) -> BCM_LeftRearDoorStatus_Convert/1
  BCM_LeftRearDoorStatus_sat/1 -> BCM_LeftRearDoorStatus_Out/1
  BCM_LeftRearDoorStatus_Ad/1 -> BCM_LeftRearDoorStatus_sat/1
  BCM_LeftRearDoorStatus_O/1 -> BCM_LeftRearDoorStatus_Ad/2
  BCM_LeftRearDoorStatus_F/1 -> BCM_LeftRearDoorStatus_Ad/1
  BCM_RightRearDoorStatuscv/1 -> BCM_RightRearDoorStatus_F/1
  BCM_RightRearDoorStatus_S/1 -> BCM_RightRearDoorStatuscv/1
  BCM_RightRearDoorStatus_L/1 -> BCM_RightRearDoorStatus_S/1
  BCM_RightRearDoorStatus_Convert/1 -> BCM_RightRearDoorStatus_L/1
  BCM_RightRearDoorStatus_Sub/1(Out1) -> BCM_RightRearDoorStatus_Convert/1
  BCM_RightRearDoorStatus_sat/1 -> BCM_RightRearDoorStatus_Out/1
  BCM_RightRearDoorStatus_Ad/1 -> BCM_RightRearDoorStatus_sat/1
  BCM_RightRearDoorStatus_O/1 -> BCM_RightRearDoorStatus_Ad/2
  BCM_RightRearDoorStatus_F/1 -> BCM_RightRearDoorStatus_Ad/1
  BCM_TrunkDoorStatuscv/1 -> BCM_TrunkDoorStatus_F/1
  BCM_TrunkDoorStatus_S/1 -> BCM_TrunkDoorStatuscv/1
  BCM_TrunkDoorStatus_L/1 -> BCM_TrunkDoorStatus_S/1
  BCM_TrunkDoorStatus_Convert/1 -> BCM_TrunkDoorStatus_L/1
  BCM_TrunkDoorStatus_Sub/1(Out1) -> BCM_TrunkDoorStatus_Convert/1
  BCM_TrunkDoorStatus_sat/1 -> BCM_TrunkDoorStatus_Out/1
  BCM_TrunkDoorStatus_Ad/1 -> BCM_TrunkDoorStatus_sat/1
  BCM_TrunkDoorStatus_O/1 -> BCM_TrunkDoorStatus_Ad/2
  BCM_TrunkDoorStatus_F/1 -> BCM_TrunkDoorStatus_Ad/1
  BCM_HoodStatuscv/1 -> BCM_HoodStatus_F/1
  BCM_HoodStatus_S/1 -> BCM_HoodStatuscv/1
  BCM_HoodStatus_L/1 -> BCM_HoodStatus_S/1
  BCM_HoodStatus_Convert/1 -> BCM_HoodStatus_L/1
  BCM_HoodStatus_Sub/1(Out1) -> BCM_HoodStatus_Convert/1
  Demux/3 -> BCM_DriverDoorStatus_Sub/1(In1), BCM_HoodStatus_Sub/1(In1), BCM_RightRearDoorStatus_Sub/1(In1), BCM_TrunkDoorStatus_Sub/1(In1), BCM_LeftRearDoorStatus_Sub/1(In1), BCM_PassengerDoorStatus_Sub/1(In1)
  BCM_HoodStatus_sat/1 -> BCM_HoodStatus_Out/1
  BCM_HoodStatus_Ad/1 -> BCM_HoodStatus_sat/1
  BCM_HoodStatus_O/1 -> BCM_HoodStatus_Ad/2
  BCM_HoodStatus_F/1 -> BCM_HoodStatus_Ad/1
  BCM_TurnIndicatorLeftcv/1 -> BCM_TurnIndicatorLeft_F/1
  BCM_TurnIndicatorLeft_S/1 -> BCM_TurnIndicatorLeftcv/1
  BCM_TurnIndicatorLeft_L/1 -> BCM_TurnIndicatorLeft_S/1
  BCM_TurnIndicatorLeft_Convert/1 -> BCM_TurnIndicatorLeft_L/1
  BCM_TurnIndicatorLeft_Sub/1(Out1) -> BCM_TurnIndicatorLeft_Convert/1
  BCM_TurnIndicatorLeft_sat/1 -> BCM_TurnIndicatorLeft_Out/1
  BCM_TurnIndicatorLeft_Ad/1 -> BCM_TurnIndicatorLeft_sat/1
  BCM_TurnIndicatorLeft_O/1 -> BCM_TurnIndicatorLeft_Ad/2
  BCM_TurnIndicatorLeft_F/1 -> BCM_TurnIndicatorLeft_Ad/1
  BCM_TurnIndicatorRightcv/1 -> BCM_TurnIndicatorRight_F/1
  BCM_TurnIndicatorRight_S/1 -> BCM_TurnIndicatorRightcv/1
  BCM_TurnIndicatorRight_L/1 -> BCM_TurnIndicatorRight_S/1
  BCM_TurnIndicatorRight_Convert/1 -> BCM_TurnIndicatorRight_L/1
  BCM_TurnIndicatorRight_Sub/1(Out1) -> BCM_TurnIndicatorRight_Convert/1
  BCM_TurnIndicatorRight_sat/1 -> BCM_TurnIndicatorRight_Out/1
  BCM_TurnIndicatorRight_Ad/1 -> BCM_TurnIndicatorRight_sat/1
  BCM_TurnIndicatorRight_O/1 -> BCM_TurnIndicatorRight_Ad/2
  BCM_TurnIndicatorRight_F/1 -> BCM_TurnIndicatorRight_Ad/1
  BCM_FrontWashStatuscv/1 -> BCM_FrontWashStatus_F/1
  BCM_FrontWashStatus_S/1 -> BCM_FrontWashStatuscv/1
  BCM_FrontWashStatus_L/1 -> BCM_FrontWashStatus_S/1
  BCM_FrontWashStatus_Convert/1 -> BCM_FrontWashStatus_L/1
  BCM_FrontWashStatus_Sub/1(Out1) -> BCM_FrontWashStatus_Convert/1
  Demux/2 -> BCM_TurnIndicatorLeft_Sub/1(In1), BCM_TurnIndicatorRight_Sub/1(In1), BCM_FrontWashStatus_Sub/1(In1)
  BCM_FrontWashStatus_sat/1 -> BCM_FrontWashStatus_Out/1
  BCM_FrontWashStatus_Ad/1 -> BCM_FrontWashStatus_sat/1
  BCM_FrontWashStatus_O/1 -> BCM_FrontWashStatus_Ad/2
  BCM_FrontWashStatus_F/1 -> BCM_FrontWashStatus_Ad/1
  Demux/4 -> ?

== system VCU_CS75_12_27_test_log/长安CS75底盘程序，20ms一次/Input/CAN1_Rx/BCM_328/ReceiveMessages/Subsystem/BCM_1 ==
  input : Inport
  Demux : Demux  Outputs=8
  LCM_DRLSts_Ad : Sum
  LCM_DRLSts_Convert : DataTypeConversion  OutDataTypeStr=uint32
  LCM_DRLSts_F : Gain
  LCM_DRLSts_L : simulink/Logic and Bit Operations/Bitwise Operator  logicop=AND  UseBitMask=on  BitMask=192  BitMaskRealWorld=Stored Integer
  LCM_DRLSts_O : Constant  Value=0  OutDataTypeStr=single
  LCM_DRLSts_S : ArithShift  BitShiftNumber=6
  LCM_DRLSts_Sub : Subsystem
  LCM_DRLSts_sat : Saturate  UpperLimit=0  LowerLimit=0
  LCM_DRLStscv : DataTypeConversion
  LCM_DriveMode_Ad : Sum
  LCM_DriveMode_Convert : DataTypeConversion  OutDataTypeStr=uint32
  LCM_DriveMode_F : Gain
  LCM_DriveMode_L : simulink/Logic and Bit Operations/Bitwise Operator  logicop=AND  UseBitMask=on  BitMask=192  BitMaskRealWorld=Stored Integer
  LCM_DriveMode_O : Constant  Value=0  OutDataTypeStr=single
  LCM_DriveMode_S : ArithShift  BitShiftNumber=6
  LCM_DriveMode_Sub : Subsystem
  LCM_DriveMode_sat : Saturate  UpperLimit=0  LowerLimit=0
  LCM_DriveModecv : DataTypeConversion
  LCM_LASSwitch_Ad : Sum
  LCM_LASSwitch_Convert : DataTypeConversion  OutDataTypeStr=uint32
  LCM_LASSwitch_F : Gain
  LCM_LASSwitch_L : simulink/Logic and Bit Operations/Bitwise Operator  logicop=AND  UseBitMask=on  BitMask=3  BitMaskRealWorld=Stored Integer
  LCM_LASSwitch_O : Constant  Value=0  OutDataTypeStr=single
  LCM_LASSwitch_S : ArithShift
  LCM_LASSwitch_Sub : Subsystem
  LCM_LASSwitch_sat : Saturate  UpperLimit=3  LowerLimit=0
  LCM_LASSwitchcv : DataTypeConversion
  LCM_RearLeftTuningLightFaultSts_Ad : Sum
  LCM_RearLeftTuningLightFaultSts_Convert : DataTypeConversion  OutDataTypeStr=uint32
  LCM_RearLeftTuningLightFaultSts_F : Gain
  LCM_RearLeftTuningLightFaultSts_L : simulink/Logic and Bit Operations/Bitwise Operator  logicop=AND  UseBitMask=on  BitMask=128  BitMaskRealWorld=Stored Integer
  LCM_RearLeftTuningLightFaultSts_O : Constant  Value=0  OutDataTypeStr=single
  LCM_RearLeftTuningLightFaultSts_S : ArithShift  BitShiftNumber=7
  LCM_RearLeftTuningLightFaultSts_Sub : Subsystem
  LCM_RearLeftTuningLightFaultSts_sat : Saturate  UpperLimit=0  LowerLimit=0
  LCM_RearLeftTuningLightFaultStscv : DataTypeConversion
  LCM_RearRightTuningLightFaultSts_Ad : Sum
  LCM_RearRightTuningLightFaultSts_Convert : DataTypeConversion  OutDataTypeStr=uint32
  LCM_RearRightTuningLightFaultSts_F : Gain
  LCM_RearRightTuningLightFaultSts_L : simulink/Logic and Bit Operations/Bitwise Operator  logicop=AND  UseBitMask=on  BitMask=128  BitMaskRealWorld=Stored Integer
  LCM_RearRightTuningLightFaultSts_O : Constant  Value=0  OutDataTypeStr=single
  LCM_RearRightTuningLightFaultSts_S : ArithShift  BitShiftNumber=7
  LCM_RearRightTuningLightFaultSts_Sub : Subsystem
  LCM_RearRightTuningLightFaultSts_sat : Saturate  UpperLimit=0  LowerLimit=0
  LCM_RearRightTuningLightFaultStscv : DataTypeConversion
  LCM_ReverseLightSts_Ad : Sum
  LCM_ReverseLightSts_Convert : DataTypeConversion  OutDataTypeStr=uint32
  LCM_ReverseLightSts_F : Gain
  LCM_ReverseLightSts_L : simulink/Logic and Bit Operations/Bitwise Operator  logicop=AND  UseBitMask=on  BitMask=192  BitMaskRealWorld=Stored Integer
  LCM_ReverseLightSts_O : Constant  Value=0  OutDataTypeStr=single
  LCM_ReverseLightSts_S : ArithShift  BitShiftNumber=6
  LCM_ReverseLightSts_Sub : Subsystem
  LCM_ReverseLightSts_sat : Saturate  UpperLimit=0  LowerLimit=0
  LCM_ReverseLightStscv : DataTypeConversion
  LCM_DriveMode_Out : Outport
  LCM_DRLSts_Out : Outport  Port=2
  LCM_LASSwitch_Out : Outport  Port=3
  LCM_RearRightTuningLightFaultSts_Out : Outport  Port=4
  LCM_RearLeftTuningLightFaultSts_Out : Outport  Port=5
  LCM_ReverseLightSts_Out : Outport  Port=6
  wires:
  input/1 -> Demux/1
  LCM_ReverseLightStscv/1 -> LCM_ReverseLightSts_F/1
  LCM_ReverseLightSts_S/1 -> LCM_ReverseLightStscv/1
  LCM_ReverseLightSts_L/1 -> LCM_ReverseLightSts_S/1
  LCM_ReverseLightSts_Convert/1 -> LCM_ReverseLightSts_L/1
  LCM_ReverseLightSts_Sub/1(Out1) -> LCM_ReverseLightSts_Convert/1
  Demux/6 -> LCM_ReverseLightSts_Sub/1(In1)
  LCM_ReverseLightSts_sat/1 -> LCM_ReverseLightSts_Out/1
  LCM_ReverseLightSts_Ad/1 -> LCM_ReverseLightSts_sat/1
  LCM_ReverseLightSts_O/1 -> LCM_ReverseLightSts_Ad/2
  LCM_ReverseLightSts_F/1 -> LCM_ReverseLightSts_Ad/1
  LCM_RearLeftTuningLightFaultStscv/1 -> LCM_RearLeftTuningLightFaultSts_F/1
  LCM_RearLeftTuningLightFaultSts_S/1 -> LCM_RearLeftTuningLightFaultStscv/1
  LCM_RearLeftTuningLightFaultSts_L/1 -> LCM_RearLeftTuningLightFaultSts_S/1
  LCM_RearLeftTuningLightFaultSts_Convert/1 -> LCM_RearLeftTuningLightFaultSts_L/1
  LCM_RearLeftTuningLightFaultSts_Sub/1(Out1) -> LCM_RearLeftTuningLightFaultSts_Convert/1
  Demux/5 -> LCM_RearLeftTuningLightFaultSts_Sub/1(In1)
  LCM_RearLeftTuningLightFaultSts_sat/1 -> LCM_RearLeftTuningLightFaultSts_Out/1
  LCM_RearLeftTuningLightFaultSts_Ad/1 -> LCM_RearLeftTuningLightFaultSts_sat/1
  LCM_RearLeftTuningLightFaultSts_O/1 -> LCM_RearLeftTuningLightFaultSts_Ad/2
  LCM_RearLeftTuningLightFaultSts_F/1 -> LCM_RearLeftTuningLightFaultSts_Ad/1
  LCM_RearRightTuningLightFaultStscv/1 -> LCM_RearRightTuningLightFaultSts_F/1
  LCM_RearRightTuningLightFaultSts_S/1 -> LCM_RearRightTuningLightFaultStscv/1
  LCM_RearRightTuningLightFaultSts_L/1 -> LCM_RearRightTuningLightFaultSts_S/1
  LCM_RearRightTuningLightFaultSts_Convert/1 -> LCM_RearRightTuningLightFaultSts_L/1
  LCM_RearRightTuningLightFaultSts_Sub/1(Out1) -> LCM_RearRightTuningLightFaultSts_Convert/1
  Demux/4 -> LCM_RearRightTuningLightFaultSts_Sub/1(In1)
  LCM_RearRightTuningLightFaultSts_sat/1 -> LCM_RearRightTuningLightFaultSts_Out/1
  LCM_RearRightTuningLightFaultSts_Ad/1 -> LCM_RearRightTuningLightFaultSts_sat/1
  LCM_RearRightTuningLightFaultSts_O/1 -> LCM_RearRightTuningLightFaultSts_Ad/2
  LCM_RearRightTuningLightFaultSts_F/1 -> LCM_RearRightTuningLightFaultSts_Ad/1
  LCM_LASSwitchcv/1 -> LCM_LASSwitch_F/1
  LCM_LASSwitch_S/1 -> LCM_LASSwitchcv/1
  LCM_LASSwitch_L/1 -> LCM_LASSwitch_S/1
  LCM_LASSwitch_Convert/1 -> LCM_LASSwitch_L/1
  LCM_LASSwitch_Sub/1(Out1) -> LCM_LASSwitch_Convert/1
  Demux/3 -> LCM_LASSwitch_Sub/1(In1)
  LCM_LASSwitch_sat/1 -> LCM_LASSwitch_Out/1
  LCM_LASSwitch_Ad/1 -> LCM_LASSwitch_sat/1
  LCM_LASSwitch_O/1 -> LCM_LASSwitch_Ad/2
  LCM_LASSwitch_F/1 -> LCM_LASSwitch_Ad/1
  LCM_DRLStscv/1 -> LCM_DRLSts_F/1
  LCM_DRLSts_S/1 -> LCM_DRLStscv/1
  LCM_DRLSts_L/1 -> LCM_DRLSts_S/1
  LCM_DRLSts_Convert/1 -> LCM_DRLSts_L/1
  LCM_DRLSts_Sub/1(Out1) -> LCM_DRLSts_Convert/1
  Demux/2 -> LCM_DRLSts_Sub/1(In1)
  LCM_DRLSts_sat/1 -> LCM_DRLSts_Out/1
  LCM_DRLSts_Ad/1 -> LCM_DRLSts_sat/1
  LCM_DRLSts_O/1 -> LCM_DRLSts_Ad/2
  LCM_DRLSts_F/1 -> LCM_DRLSts_Ad/1
  LCM_DriveModecv/1 -> LCM_DriveMode_F/1
  LCM_DriveMode_S/1 -> LCM_DriveModecv/1
  LCM_DriveMode_L/1 -> LCM_DriveMode_S/1
  LCM_DriveMode_Convert/1 -> LCM_DriveMode_L/1
  LCM_DriveMode_Sub/1(Out1) -> LCM_DriveMode_Convert/1
  Demux/1 -> LCM_DriveMode_Sub/1(In1)
  LCM_DriveMode_sat/1 -> LCM_DriveMode_Out/1
  LCM_DriveMode_Ad/1 -> LCM_DriveMode_sat/1
  LCM_DriveMode_O/1 -> LCM_DriveMode_Ad/2
  LCM_DriveMode_F/1 -> LCM_DriveMode_Ad/1

== system VCU_CS75_12_27_test_log/长安CS75底盘程序，20ms一次/Input/CAN1_Rx/BCM_348/ReceiveMessages/Subsystem/BCM_1 ==
  input : Inport
  BCM_DriveMode_Ad : Sum
  BCM_DriveMode_Convert : DataTypeConversion  OutDataTypeStr=uint32
  BCM_DriveMode_F : Gain
  BCM_DriveMode_L : simulink/Logic and Bit Operations/Bitwise Operator  logicop=AND  UseBitMask=on  BitMask=6  BitMaskRealWorld=Stored Integer
  BCM_DriveMode_O : Constant  Value=0  OutDataTypeStr=single
  BCM_DriveMode_S : ArithShift  BitShiftNumber=1
  BCM_DriveMode_Sub : Subsystem
  BCM_DriveMode_sat : Saturate  UpperLimit=3  LowerLimit=0
  BCM_DriveModecv : DataTypeConversion
  BCM_LockSignal_Ad : Sum
  BCM_LockSignal_Convert : DataTypeConversion  OutDataTypeStr=uint32
  BCM_LockSignal_F : Gain
  BCM_LockSignal_L : simulink/Logic and Bit Operations/Bitwise Operator  logicop=AND  UseBitMask=on  BitMask=24  BitMaskRealWorld=Stored Integer
  BCM_LockSignal_O : Constant  Value=0  OutDataTypeStr=single
  BCM_LockSignal_S : ArithShift  BitShiftNumber=3
  BCM_LockSignal_Sub : Subsystem
  BCM_LockSignal_sat : Saturate  UpperLimit=3  LowerLimit=0
  BCM_LockSignalcv : DataTypeConversion
  BCM_UnlockSignal_Ad : Sum
  BCM_UnlockSignal_Convert : DataTypeConversion  OutDataTypeStr=uint32
  BCM_UnlockSignal_F : Gain
  BCM_UnlockSignal_L : simulink/Logic and Bit Operations/Bitwise Operator  logicop=AND  UseBitMask=on  BitMask=96  BitMaskRealWorld=Stored Integer
  BCM_UnlockSignal_O : Constant  Value=0  OutDataTypeStr=single
  BCM_UnlockSignal_S : ArithShift  BitShiftNumber=5
  BCM_UnlockSignal_Sub : Subsystem
  BCM_UnlockSignal_sat : Saturate  UpperLimit=3  LowerLimit=0
  BCM_UnlockSignalcv : DataTypeConversion
  Demux : Demux  Outputs=8
  BCM_DriveMode_Out : Outport
  BCM_LockSignal_Out : Outport  Port=2
  BCM_UnlockSignal_Out : Outport  Port=3
  wires:
  input/1 -> Demux/1
  BCM_UnlockSignalcv/1 -> BCM_UnlockSignal_F/1
  BCM_UnlockSignal_S/1 -> BCM_UnlockSignalcv/1
  BCM_UnlockSignal_L/1 -> BCM_UnlockSignal_S/1
  BCM_UnlockSignal_Convert/1 -> BCM_UnlockSignal_L/1
  BCM_UnlockSignal_Sub/1(Out1) -> BCM_UnlockSignal_Convert/1
  BCM_UnlockSignal_sat/1 -> BCM_UnlockSignal_Out/1
  BCM_UnlockSignal_Ad/1 -> BCM_UnlockSignal_sat/1
  BCM_UnlockSignal_O/1 -> BCM_UnlockSignal_Ad/2
  BCM_UnlockSignal_F/1 -> BCM_UnlockSignal_Ad/1
  BCM_LockSignalcv/1 -> BCM_LockSignal_F/1
  BCM_LockSignal_S/1 -> BCM_LockSignalcv/1
  BCM_LockSignal_L/1 -> BCM_LockSignal_S/1
  BCM_LockSignal_Convert/1 -> BCM_LockSignal_L/1
  BCM_LockSignal_Sub/1(Out1) -> BCM_LockSignal_Convert/1
  BCM_LockSignal_sat/1 -> BCM_LockSignal_Out/1
  BCM_LockSignal_Ad/1 -> BCM_LockSignal_sat/1
  BCM_LockSignal_O/1 -> BCM_LockSignal_Ad/2
  BCM_LockSignal_F/1 -> BCM_LockSignal_Ad/1
  BCM_DriveModecv/1 -> BCM_DriveMode_F/1
  BCM_DriveMode_S/1 -> BCM_DriveModecv/1
  BCM_DriveMode_L/1 -> BCM_DriveMode_S/1
  BCM_DriveMode_Convert/1 -> BCM_DriveMode_L/1
  BCM_DriveMode_Sub/1(Out1) -> BCM_DriveMode_Convert/1
  Demux/6 -> BCM_UnlockSignal_Sub/1(In1), BCM_LockSignal_Sub/1(In1), BCM_DriveMode_Sub/1(In1)
  BCM_DriveMode_sat/1 -> BCM_DriveMode_Out/1
  BCM_DriveMode_Ad/1 -> BCM_DriveMode_sat/1
  BCM_DriveMode_O/1 -> BCM_DriveMode_Ad/2
  BCM_DriveMode_F/1 -> BCM_DriveMode_Ad/1
